simulink model "ssc_auto_ev_20b"  (R2020b)
settings: Solver=VariableStepAuto  StartTime=0.0  StopTime=200  RelTol=1e-3  AbsTol=1e-3
PreLoadFcn:
  | % Simulation parameters
  | dt = 0.01;
  | 
  | % Battery cell parameters
  | ssc_lithium_cell_1RC_ini
  | Nseries = 100;
  | Nparallel = 10;
  | 
  | % Motor parameters
  | max_torque = 220;
  | max_power = 80e3;
  | 
  | % Vehicle parameters
  | vehicle_mass = 4000;
  | wheel_radius = 0.35;
  | area = 5;
  | drag_coefficient = 0.25;
  | air_density = 1.225;
  | gravity = 9.81;
  | rolling_res_ratio = 0.015;
  | 
  | % Differential drive parameters
  | gear_ratio = 12;
  | 
  | % Simplified braking system parameters
  | force_max_pedal = 500;
  | braking_torque_to_pedal_force_ratio = -16;
  | 
  | % Vehicle controller parameters
  | hill_hold_max_speed = 0.5;
  | 
  | % Water properties for cooling circuit
  | load WaterProperties
  | 
  | % Input signals for Signal Editor block
  | load ssc_auto_ev_Inputs
values from neighbouring files (symbols this model uses):
  C1_LUT = [1913.6 4625.7 23306 10736 18036 12251 9022.9 12447 18872 40764 18721 33630 ... (21 elements, 7x3)]    [ssc_auto_ev_param.mat]
  Capacity_LUT = [28.0081 27.625 27.6392]    [ssc_auto_ev_param.mat]
  cell_Cp_heat = 810.5328    [ssc_auto_ev_param.mat]
  cell_mass = 1    [ssc_auto_ev_param.mat]
  Em_LUT = [3.4966 3.5519 3.6183 3.7066 3.9131 4.0748 4.1923 3.5057 3.566 3.6337 3.7127 3.9259 ... (21 elements, 7x3)]    [ssc_auto_ev_param.mat]
  Qe_init = 15.6845    [ssc_auto_ev_param.mat]
  R0_LUT = [0.0117 0.011 0.0114 0.0107 0.0107 0.0113 0.0116 0.0085 0.0085 0.0087 0.0082 0.0083 ... (21 elements, 7x3)]    [ssc_auto_ev_param.mat]
  R1_LUT = [0.0109 0.0069 0.0047 0.0034 0.0033 0.0033 0.0028 0.0029 0.0024 0.0026 0.0016 0.0023 ... (21 elements, 7x3)]    [ssc_auto_ev_param.mat]
  SOC_LUT = [0 0.1 0.25 0.5 0.75 0.9 1]    [ssc_auto_ev_param.mat]
  T_init = 293.15    [ssc_auto_ev_param.mat]
  Temperature_LUT = [278.15 293.15 313.15]    [ssc_auto_ev_param.mat]
undefined symbols (not defined in the file or in its folder): DiscIntNeverNeededParam, K, Lambda, tau, x0
libraries: fl_lib x656, nesl_utility x86, simulink x21, LiBatteryElements_lib x16, SignalEditorBlockLib x4, simulink_extras x4
(part 9 of 13)

== system ssc_auto_ev_20b/Step 3: Ungroup and Redraw/Motor Drive/DC Motor2 ==
  Inertia : fl_lib/Mechanical/Rotational Elements/Inertia  inertia=0.01 kg*m^2  num_ports=foundation.enum.numPorts2.one  w_specify=off  w_priority=High  w=0 rad/s  w_nominal_specify=off  w_nominal_unit=rad/s  w_nominal_value=1  t_specify=off  t_priority=High  t=0 N*m  t_nominal_specify=off  t_nominal_unit=N*m  t_nominal_value=1
      settings: SourceProductBaseCode=PW,SS,VE
  Rotational Electromechanical Converter : fl_lib/Electrical/Electrical Elements/Rotational Electromechanical Converter  K=1 N*m/A  i_specify=off  i_priority=High  i=0 A  i_nominal_specify=off  i_nominal_unit=A  i_nominal_value=1  v_specify=off  v_priority=High  v=0 V  v_nominal_specify=off  v_nominal_unit=V  v_nominal_value=1  t_specify=off  t_priority=High  t=0 N*m  t_nominal_specify=off  t_nominal_unit=N*m  t_nominal_value=1  w_specify=off  w_priority=High  w=0 rad/s  w_nominal_specify=off  w_nominal_unit=rad/s  w_nominal_value=1
      settings: SourceProductBaseCode=PW,SS,VE
  Thermal Resistor : fl_lib/Electrical/Electrical Elements/Thermal Resistor  R0=1 Ohm  T0=298.15 K  alpha=50e-6 1/K  tc=30 s  K_d=100 W/K  T_specify=off  T_priority=High  T=300 K  T_nominal_specify=off  T_nominal_unit=K  T_nominal_value=1
      settings: SourceProductBaseCode=PW,SS,VE  InternalSimscapePortConfiguration="{\"Bottom\":[],\"Left\":[{\"id\":\"H\",\"label\":\"H\",\"type\":\"foundation.thermal.thermal\"},{\"id\":\"p\",\"label\":\"+\",\"type\":\"foundation.electrical.electrical\"}],\"Right\":[{\"id\":\"n\",\"label\":\"-\",\"type\":\"foundation.electrical.electrical\"}],\"Top\":[]}"
  V+ : PMIOPort  Side=Left
  R : PMIOPort  Port=2  Side=Right
  C : PMIOPort  Port=3  Side=Right
  V- : PMIOPort  Port=4  Side=Left
  H : PMIOPort  Port=5  Side=Left
  connections:
  Thermal Resistor/RConn1 -- Rotational Electromechanical Converter/LConn1
  V-/RConn1 -- Rotational Electromechanical Converter/RConn1
  Thermal Resistor/LConn2 -- V+/RConn1
  Rotational Electromechanical Converter/LConn2 -- Inertia/LConn1 -- R/RConn1
  Rotational Electromechanical Converter/RConn2 -- C/RConn1
  H/RConn1 -- Thermal Resistor/LConn1

== system ssc_auto_ev_20b/Step 3: Ungroup and Redraw/Motor Drive/Motor Torque Controller 1 (System-Level Representation) ==
  Controlled Current Source : fl_lib/Electrical/Electrical Sources/Controlled Current Source
      settings: SourceProductBaseCode=PW,SS,VE
  +1 : PMIOPort  Side=Right
  +2 : PMIOPort  Port=2  Side=Left
  -1 : PMIOPort  Port=3  Side=Right
  -2 : PMIOPort  Port=4  Side=Left
  iRef : PMIOPort  Port=5  Side=Left
  connections:
  iRef/RConn1 -- Controlled Current Source/RConn1
  -2/RConn1 -- -1/RConn1
  Controlled Current Source/LConn1 -- +2/RConn1
  Controlled Current Source/RConn2 -- +1/RConn1

== system ssc_auto_ev_20b/Step 3: Ungroup and Redraw/Motor Drive/Motor Torque Controller 1 (System-Level Representation)1 ==
  Controlled Current Source : fl_lib/Electrical/Electrical Sources/Controlled Current Source
      settings: SourceProductBaseCode=PW,SS,VE
  +1 : PMIOPort  Side=Right
  +2 : PMIOPort  Port=2  Side=Left
  -1 : PMIOPort  Port=3  Side=Right
  -2 : PMIOPort  Port=4  Side=Left
  iRef : PMIOPort  Port=5  Side=Left
  connections:
  Controlled Current Source/RConn2 -- +1/RConn1
  Controlled Current Source/LConn1 -- +2/RConn1
  -2/RConn1 -- -1/RConn1
  iRef/RConn1 -- Controlled Current Source/RConn1

== system ssc_auto_ev_20b/Step 3: Ungroup and Redraw/Motor Drive/Sensing wMotor ==
  PS-Simulink Converter : nesl_utility/PS-Simulink Converter  PhysicalDomain=network_engine_domain  SubClassName=ps_output  LeftPortType=input  RightPortType=output  PseudoPeriodic=off  Frequencies=[]  Unit=rad/s  AffineConversion=off
      settings: SourceProductBaseCode=SS,PW,VE
  PS : PMIOPort  Side=Left
  SL : Outport  VectorParamsAs1DForOutWhenUnconnected=off
  wires:
  PS-Simulink Converter/1 -> SL/1
  connections:
  PS/RConn1 -- PS-Simulink Converter/LConn1

== system ssc_auto_ev_20b/Step 3: Ungroup and Redraw/Port 1 Interface/Interface ==
  through1 : Inport
  through2 : Inport  Port=2
  Continuous : Subsystem  VariantControl=Continuous
  Discrete : Subsystem  VariantControl=Discrete
  across2 : Outport
  across1 : Outport  Port=2

== system ssc_auto_ev_20b/Step 3: Ungroup and Redraw/Port 1 Interface1/Interface ==
  through1 : Inport
  through2 : Inport  Port=2
  Continuous : Subsystem  VariantControl=Continuous
  Discrete : Subsystem  VariantControl=Discrete
  across2 : Outport
  across1 : Outport  Port=2

== system ssc_auto_ev_20b/Step 3: Ungroup and Redraw/Port 1 Interface2/Interface ==
  through1 : Inport
  through2 : Inport  Port=2
  Continuous : Subsystem  VariantControl=Continuous
  Discrete : Subsystem  VariantControl=Discrete
  across2 : Outport
  across1 : Outport  Port=2

== system ssc_auto_ev_20b/Step 3: Ungroup and Redraw/Port 1 Interface3/Interface ==
  through1 : Inport
  across2 : Inport  Port=2
  Continuous : Subsystem  VariantControl=Continuous
  Discrete : Subsystem  VariantControl=Discrete
  through2 : Outport
  across1 : Outport  Port=2

== system ssc_auto_ev_20b/Step 3: Ungroup and Redraw/Vehicle Dynamics/Brake Torque ==
  Pedal : Inport
  Force for max pedal deflection : Gain  Gain=force_max_pedal
  Ideal Torque Source : fl_lib/Mechanical/Mechanical Sources/Ideal Torque Source
      settings: SourceProductBaseCode=PW,SS,VE
  MRRef : fl_lib/Mechanical/Rotational Elements/Mechanical Rotational Reference
      settings: SourceProductBaseCode=PW,SS,VE
  Motion Sensor : fl_lib/Mechanical/Mechanical Sensors/Ideal Rotational Motion Sensor  wrap_angle=simscape.enum.onoff.off  offset=0 rad
      settings: SourceProductBaseCode=PW,SS,VE
  PS Product : fl_lib/Physical Signals/Functions/PS Product
      settings: SourceProductBaseCode=PW,SS,VE
  Simulink-PS Converter1 : nesl_utility/Simulink-PS Converter  PhysicalDomain=network_engine_domain  SubClassName=ps_input  LeftPortType=input  RightPortType=output  PseudoPeriodic=off  Frequencies=[]  NoiseDistribution=none  NoiseParameters=[]  Unit=N*m  AffineConversion=off  FilteringAndDerivatives=zero  SimscapeFilterOrder=1  InputFilterTimeConstant=0.001  UdotUserProvided=1
      settings: SourceProductBaseCode=SS,PW,VE
  Smooth Sign : Subsystem
  Torque per unit brake pedal force : Gain  Gain=braking_torque_to_pedal_force_ratio
  R : PMIOPort  Side=Right
  wires:
  Torque per unit brake pedal force/1 -> Simulink-PS Converter1/1
  Pedal/1 -> Force for max pedal deflection/1
  Force for max pedal deflection/1 -> Torque per unit brake pedal force/1
  connections:
  Smooth Sign/RConn1 -- PS Product/LConn1
  Motion Sensor/RConn1 -- MRRef/LConn1 -- Ideal Torque Source/RConn2
  Ideal Torque Source/LConn1 -- Motion Sensor/LConn1 -- R/RConn1
  PS Product/RConn1 -- Ideal Torque Source/RConn1
  PS Product/LConn2 -- Simulink-PS Converter1/RConn1
  Smooth Sign/LConn1 -- Motion Sensor/RConn2

== system ssc_auto_ev_20b/Step 3: Ungroup and Redraw/Vehicle Dynamics/Drag and Gravity ==
  beta : Inport
  vW : Inport  Port=2
  " M*g " : fl_lib/Physical Signals/Functions/PS Gain  gain=vehicle_mass*gravity kg*m/s^2
      settings: SourceProductBaseCode=PW,SS,VE
  " tanh(u) " : fl_lib/Physical Signals/Functions/PS Math Function  fcn_choice=foundation.enum.math_function.tanh
      settings: SourceProductBaseCode=PW,SS,VE
  -1 : fl_lib/Physical Signals/Functions/PS Gain  gain=-1
      settings: SourceProductBaseCode=PW,SS,VE
  0.5*Cd*density*area : fl_lib/Physical Signals/Functions/PS Gain  gain=0.5*drag_coefficient*air_density*area kg/m^3*m^2
      settings: SourceProductBaseCode=PW,SS,VE
  1s/m : fl_lib/Physical Signals/Functions/PS Gain  gain=1 1/(m/s)
      settings: SourceProductBaseCode=PW,SS,VE
  M*g : fl_lib/Physical Signals/Functions/PS Gain  gain=vehicle_mass*gravity kg*m/s^2
      settings: SourceProductBaseCode=PW,SS,VE
  PS Add : fl_lib/Physical Signals/Functions/PS Add
      settings: SourceProductBaseCode=PW,SS,VE
  PS Gain : fl_lib/Physical Signals/Functions/PS Gain  gain=1 1/(m/s)
      settings: SourceProductBaseCode=PW,SS,VE
  PS Product : fl_lib/Physical Signals/Functions/PS Product
      settings: SourceProductBaseCode=PW,SS,VE
  PS Product2 : fl_lib/Physical Signals/Functions/PS Product
      settings: SourceProductBaseCode=PW,SS,VE
  PS Subtract : fl_lib/Physical Signals/Functions/PS Subtract
      settings: SourceProductBaseCode=PW,SS,VE
  Rolling resistance (fraction of normal force) : fl_lib/Physical Signals/Functions/PS Gain  gain=rolling_res_ratio
      settings: SourceProductBaseCode=PW,SS,VE
  Simulink-PS Converter2 : nesl_utility/Simulink-PS Converter  PhysicalDomain=network_engine_domain  SubClassName=ps_input  LeftPortType=input  RightPortType=output  PseudoPeriodic=off  Frequencies=[]  NoiseDistribution=none  NoiseParameters=[]  Unit=m/s  AffineConversion=off  FilteringAndDerivatives=zero  SimscapeFilterOrder=1  InputFilterTimeConstant=0.001  UdotUserProvided=1
      settings: SourceProductBaseCode=SS,PW,VE
  Simulink-PS Converter3 : nesl_utility/Simulink-PS Converter  PhysicalDomain=network_engine_domain  SubClassName=ps_input  LeftPortType=input  RightPortType=output  PseudoPeriodic=off  Frequencies=[]  NoiseDistribution=none  NoiseParameters=[]  Unit=deg  AffineConversion=off  FilteringAndDerivatives=zero  SimscapeFilterOrder=1  InputFilterTimeConstant=0.001  UdotUserProvided=1
      settings: SourceProductBaseCode=SS,PW,VE
  cos(u) : fl_lib/Physical Signals/Functions/PS Math Function  fcn_choice=foundation.enum.math_function.cos
      settings: SourceProductBaseCode=PW,SS,VE
  sin(u) : fl_lib/Physical Signals/Functions/PS Math Function  fcn_choice=foundation.enum.math_function.sin
      settings: SourceProductBaseCode=PW,SS,VE
  tanh(u) : fl_lib/Physical Signals/Functions/PS Math Function  fcn_choice=foundation.enum.math_function.tanh
      settings: SourceProductBaseCode=PW,SS,VE
  u^2 : fl_lib/Physical Signals/Functions/PS Math Function  fcn_choice=foundation.enum.math_function.square
      settings: SourceProductBaseCode=PW,SS,VE
  vV : PMIOPort  Side=Left
  F : PMIOPort  Port=2  Side=Left
  F2 : PMIOPort  Port=3  Side=Left
  wires:
  beta/1 -> Simulink-PS Converter3/1
  vW/1 -> Simulink-PS Converter2/1
  connections:
  " M*g "/LConn1 -- cos(u)/RConn1
  M*g/LConn1 -- sin(u)/RConn1
  Rolling resistance (fraction of normal force)/LConn1 -- " M*g "/RConn1
  M*g/RConn1 -- PS Add/LConn1
  sin(u)/LConn1 -- Simulink-PS Converter3/RConn1 -- cos(u)/LConn1
  PS Product2/LConn2 -- 0.5*Cd*density*area/RConn1
  " tanh(u) "/LConn1 -- PS Gain/RConn1
  0.5*Cd*density*area/LConn1 -- u^2/RConn1
  " tanh(u) "/RConn1 -- PS Product2/LConn1
  u^2/LConn1 -- PS Subtract/RConn1 -- PS Gain/LConn1
  tanh(u)/LConn1 -- 1s/m/RConn1
  PS Product/LConn1 -- tanh(u)/RConn1
  -1/RConn1 -- F2/RConn1
  PS Add/RConn1 -- -1/LConn1
  PS Product/RConn1 -- PS Add/LConn2
  PS Product/LConn2 -- Rolling resistance (fraction of normal force)/RConn1
  PS Product2/RConn1 -- F/RConn1
  Simulink-PS Converter2/RConn1 -- PS Subtract/LConn2
  PS Subtract/LConn1 -- 1s/m/LConn1 -- vV/RConn1

== system ssc_auto_ev_20b/Step 3: Ungroup and Redraw/Vehicle Dynamics/Sensing Speed ==
  MTRef : fl_lib/Mechanical/Translational Elements/Mechanical Translational Reference
      settings: SourceProductBaseCode=PW,SS,VE
  Motion Sensor : fl_lib/Mechanical/Mechanical Sensors/Ideal Translational Motion Sensor  offset=0 m
      settings: SourceProductBaseCode=PW,SS,VE
  R : PMIOPort  Side=Left
  w : PMIOPort  Port=2  Side=Right
  connections:
  R/RConn1 -- Motion Sensor/LConn1
  MTRef/LConn1 -- Motion Sensor/RConn1
  Motion Sensor/RConn2 -- w/RConn1

== system ssc_auto_ev_20b/Step 3: Ungroup and Redraw/Vehicle Control/Cruise Control ==
  Enable : Inport
  Disable : Inport  Port=2
  wMeas : Inport  Port=3
  Brake sw : Inport  Port=4
  Capture speed : Subsystem  TreatAsAtomicUnit=on
  Data Type Conversion1 : DataTypeConversion  OutDataTypeStr=boolean
  J-K Flip-Flop : simulink_extras/Flip Flops/J-K Flip-Flop  initial_condition=0
  Logical Operator : Logic  Operator=OR  AllPortsSameDT=off  OutDataTypeStr=boolean
  Pulse Generator : DiscretePulseGenerator  Period=10  PulseWidth=5  SampleTime=0.01
  Speed Controller : Subsystem  mask(P+I motor speed controller){Kp=100, Ki=100, trqMax=max_torque, ts=dt}
      mask prompts: Kp "Proportional gain (Nm/(rad/s))"; Ki "Integral gain (Nm/rad)"; trqMax "Maximum torque demand"; ts "Sample time"
      mask help: Inputs wRef and wMeas are the demanded rotor speed and measured rotor speed in rad/s. The controller output is a torque demand in Nm.
  Terminator : Terminator
  trqRef : Outport  VectorParamsAs1DForOutWhenUnconnected=off
  Enabled : Outport  Port=2  VectorParamsAs1DForOutWhenUnconnected=off
  wires:
  Enable/1 -> Data Type Conversion1/1
  Pulse Generator/1 -> J-K Flip-Flop/2
  Disable/1 -> Logical Operator/1
  Speed Controller/1(trqRef) -> trqRef/1
  Brake sw/1 -> Logical Operator/2
  wMeas/1 -> Capture speed/1(In1), Speed Controller/2(wMeas)
  Logical Operator/1 -> J-K Flip-Flop/3
  J-K Flip-Flop/1 -> Enabled/1, Capture speed/Trigger
  Data Type Conversion1/1 -> J-K Flip-Flop/1
  J-K Flip-Flop/2 -> Terminator/1
  Capture speed/1(Out1) -> Speed Controller/1(wRef)

== system ssc_auto_ev_20b/Step 3: Ungroup and Redraw/Vehicle Control/Feedforward term for regenerative braking on downhill ==
  Inclin. : Inport
  " M " : Gain  Gain=vehicle_mass
  1/ratio : Gain  Gain=1/gear_ratio
  Two motors : Gain  Gain=0.5
  Wheel radius : Gain  Gain=wheel_radius
  "[-inf,0]" : Saturate  UpperLimit=0  LowerLimit=-inf
  Feedfwd trq : Outport  VectorParamsAs1DForOutWhenUnconnected=off
  wires:
  Two motors/1 -> Feedfwd trq/1
  1/ratio/1 -> Two motors/1  "Motor torque"
  "[-inf,0]"/1 -> " M "/1
  Inclin./1 -> "[-inf,0]"/1
  " M "/1 -> Wheel radius/1
  Wheel radius/1 -> 1/ratio/1  "Wheel torque"

== system ssc_auto_ev_20b/Step 3: Ungroup and Redraw/Vehicle Control/Max Power ==
  Vspd : Inport
  Abs : Abs
  Constant : Constant
  Math Function : Math  Operator=reciprocal  SignedPower=on  SaturateOnIntegerOverflow=on
  Prevent divide by zero : Switch  Criteria=u2 > Threshold  Threshold=1
  max_power : Gain  Gain=max_power
  Max Power : Outport  VectorParamsAs1DForOutWhenUnconnected=off
  wires:
  Prevent divide by zero/1 -> Math Function/1
  Constant/1 -> Prevent divide by zero/3
  Abs/1 -> Prevent divide by zero/2, Prevent divide by zero/1
  Math Function/1 -> max_power/1
  max_power/1 -> Max Power/1
  Vspd/1 -> Abs/1

== system ssc_auto_ev_20b/Step 3: Ungroup and Redraw/Vehicle Control/Torque Demand Management ==
  Brake : Inport
  Throttle : Inport  Port=2
  wMeas : Inport  Port=3
  FFbrake : Inport  Port=4
  1/ratio : Gain  Gain=1/gear_ratio
  Disable braking at low and negative speeds : Lookup_n-D  NumberOfTableDimensions=1  BreakpointsForDimension1=[-100 -1 0 5 10 100]  Table=[0 0 0 0 1 1]  InternalRulePriority=Speed  RndMeth=Simplest  InputSameDT=on
  Disable braking at low and negative speeds1 : Lookup_n-D  NumberOfTableDimensions=1  BreakpointsForDimension1=[-100 -1 0 5 10 100]  Table=[0 0 0 0 1 1]  InternalRulePriority=Speed  RndMeth=Simplest  InputSameDT=on
  Force for max pedal deflection : Gain  Gain=force_max_pedal
  Max torque demand : Gain  Gain=max_torque
  Motor torque limits2 : Saturate  UpperLimit=max_torque  LowerLimit=-max_torque
  Product : Product
  Product1 : Product
  Sum : Sum  Inputs=|++
  Sum1 : Sum  Inputs=|++
  Torque per unit brake pedal force : Gain  Gain=braking_torque_to_pedal_force_ratio
  Two motors : Gain  Gain=1/2
  wMeas1 : InportShadow  Port=3
  Dem trq : Outport  VectorParamsAs1DForOutWhenUnconnected=off
  wires:
  Motor torque limits2/1 -> Dem trq/1
  Sum1/1 -> Motor torque limits2/1
  Product1/1 -> Sum1/2
  wMeas1/1 -> Disable braking at low and negative speeds1/1
  Disable braking at low and negative speeds1/1 -> Product1/2
  FFbrake/1 -> Product1/1
  Disable braking at low and negative speeds/1 -> Product/2
  Sum/1 -> Sum1/1
  Max torque demand/1 -> Sum/1
  Brake/1 -> Force for max pedal deflection/1
  Throttle/1 -> Max torque demand/1
  Torque per unit brake pedal force/1 -> 1/ratio/1
  1/ratio/1 -> Two motors/1
  Force for max pedal deflection/1 -> Torque per unit brake pedal force/1
  wMeas/1 -> Disable braking at low and negative speeds/1
  Product/1 -> Sum/2
  Two motors/1 -> Product/1

== system ssc_auto_ev_20b/Step 4: Deployment Model/Battery @50Hz/Battery ==
  note: Scale up voltage drop to total
      | of Ns series-connected cells
  Controlled Voltage Source : fl_lib/Electrical/Electrical Sources/Controlled Voltage Source
      settings: SourceProductBaseCode=PW,SS,VE
  Electric and Thermal Model : Subsystem  Tag=PublishSubsystem
  Nseries-1 : fl_lib/Physical Signals/Functions/PS Gain  gain=Nseries-1
      settings: SourceProductBaseCode=PW,SS,VE
  PS Terminator : fl_lib/Physical Signals/Sinks/PS Terminator
      settings: SourceProductBaseCode=PW,SS,VE
  Temperature Sensor : fl_lib/Thermal/Thermal Sensors/Temperature Sensor
      settings: SourceProductBaseCode=PW,SS,VE
  Thermal Reference : fl_lib/Thermal/Thermal Elements/Thermal Reference
      settings: SourceProductBaseCode=PW,SS,VE
  Voltage Sensor : fl_lib/Electrical/Electrical Sensors/Voltage Sensor
      settings: SourceProductBaseCode=PW,SS,VE
  + : PMIOPort  Tag=PMCPort  Side=Right
  H : PMIOPort  Tag=PMCPort  Port=2  Side=Left
  - : PMIOPort  Tag=PMCPort  Port=3  Side=Left
  connections:
  PS Terminator/LConn1 -- Temperature Sensor/RConn2
  Temperature Sensor/RConn1 -- Thermal Reference/LConn1
  Controlled Voltage Source/RConn2 -- -/RConn1
  Nseries-1/RConn1 -- Controlled Voltage Source/RConn1
  +/RConn1 -- Electric and Thermal Model/RConn1 -- Voltage Sensor/LConn1
  Nseries-1/LConn1 -- Voltage Sensor/RConn1
  Electric and Thermal Model/RConn2 -- Voltage Sensor/RConn2 -- Controlled Voltage Source/LConn1
  Electric and Thermal Model/LConn1 -- Temperature Sensor/LConn1 -- H/RConn1

== system ssc_auto_ev_20b/Step 4: Deployment Model/Battery @50Hz/Port 1 Interface ==
  heat flow : Inport
  Controlled Temperature Source : fl_lib/Thermal/Thermal Sources/Controlled Temperature Source
      settings: SourceProductBaseCode=PW,SS,VE
  Heat Flow Rate Sensor : fl_lib/Thermal/Thermal Sensors/Heat Flow Rate Sensor
      settings: SourceProductBaseCode=PW,SS,VE
  Interface : Subsystem  Variant=on  VariantControlMode=label  VariantControl=Variant1  LabelModeActiveChoice=Discrete
      settings: PortSchema="{\"entries\":[{\"content\":{\"sides\":[{\"content\":{\"connectorIds\":[\"In1\",\"Out2\"]},\"type\":\"ConnectorPlacement.EquallySpacedRectSide\",\"uuid\":\"aa56821c-7799-44e3-b228-553c5b43a68d\"},{\"content\":{\"connectorIds\":[\"In2\",\"Out1\"],\"side\":\"RIGHT\"},\"type\":\"ConnectorPlacement.EquallySpacedRectSide\",\"uuid\":\"8658dee5-55e2-4f33-bdec-e6600ce27fc1\"},{\"content\":{\"connectorIds\":[],\"side\":\"TOP\"},\"type\":\"ConnectorPlacement.EquallySpacedRectSide\",\"uuid\":\"2effe9c6-8e61-4f0c-a39b-329d9ffc707d\"}]},\"type\":\"ConnectorPlacement.EquallySpacedConnector\",\"uuid\":\"c8fc8444-dfc7-49a5-9550-b957635f7d8f\"}],\"packageUris\":[\"http://schema.mathworks.com/mf0/Connector/R2020b\"],\"version\":\"1.0\"}"
  T1 : nesl_utility/Simulink-PS Converter  PhysicalDomain=network_engine_domain  SubClassName=ps_input  LeftPortType=input  RightPortType=output  PseudoPeriodic=off  Frequencies=[]  NoiseDistribution=none  NoiseParameters=[]  Unit=K  AffineConversion=off  FilteringAndDerivatives=provide  SimscapeFilterOrder=1  InputFilterTimeConstant=0.001  UdotUserProvided=0
      settings: SourceProductBaseCode=SS,PW,VE
  Thermal Reference : fl_lib/Thermal/Thermal Elements/Thermal Reference
      settings: SourceProductBaseCode=PW,SS,VE
  q1 : nesl_utility/PS-Simulink Converter  PhysicalDomain=network_engine_domain  SubClassName=ps_output  LeftPortType=input  RightPortType=output  PseudoPeriodic=off  Frequencies=[]  Unit=W  AffineConversion=off
      settings: SourceProductBaseCode=SS,PW,VE
  1 : PMIOPort  Side=Left
  temperature : Outport
  wires:
  Interface/1(across2) -> temperature/1
  q1/1 -> Interface/1(through1)
  heat flow/1 -> Interface/2(through2)
  Interface/2(across1) -> T1/1
  connections:
  Heat Flow Rate Sensor/RConn2 -- Controlled Temperature Source/LConn1
  Heat Flow Rate Sensor/LConn1 -- 1/RConn1
  q1/LConn1 -- Heat Flow Rate Sensor/RConn1
  Thermal Reference/LConn1 -- Controlled Temperature Source/RConn2
  Controlled Temperature Source/RConn1 -- T1/RConn1

== system ssc_auto_ev_20b/Step 4: Deployment Model/Battery @50Hz/Port 2 Interface3 ==
  current : Inport
  Controlled Current Source : fl_lib/Electrical/Electrical Sources/Controlled Current Source
      settings: SourceProductBaseCode=PW,SS,VE
  Electrical Reference : fl_lib/Electrical/Electrical Elements/Electrical Reference
      settings: SourceProductBaseCode=PW,SS,VE
  Electrical Reference1 : fl_lib/Electrical/Electrical Elements/Electrical Reference
      settings: SourceProductBaseCode=PW,SS,VE
  In : nesl_utility/Simulink-PS Converter  PhysicalDomain=network_engine_domain  SubClassName=ps_input  LeftPortType=input  RightPortType=output  PseudoPeriodic=off  Frequencies=[]  NoiseDistribution=none  NoiseParameters=[]  Unit=A  AffineConversion=off  FilteringAndDerivatives=zero  SimscapeFilterOrder=1  InputFilterTimeConstant=0.001  UdotUserProvided=1
      settings: SourceProductBaseCode=SS,PW,VE
  Vn : nesl_utility/PS-Simulink Converter  PhysicalDomain=network_engine_domain  SubClassName=ps_output  LeftPortType=input  RightPortType=output  PseudoPeriodic=off  Frequencies=[]  Unit=V  AffineConversion=off
      settings: SourceProductBaseCode=SS,PW,VE
  Voltage Sensor : fl_lib/Electrical/Electrical Sensors/Voltage Sensor
      settings: SourceProductBaseCode=PW,SS,VE
  2 : PMIOPort  Side=Right
  voltage : Outport
  wires:
  current/1 -> In/1
  Vn/1 -> voltage/1
  connections:
  In/RConn1 -- Controlled Current Source/RConn1
  Controlled Current Source/LConn1 -- Electrical Reference/LConn1
  Voltage Sensor/RConn1 -- Vn/LConn1
  2/RConn1 -- Controlled Current Source/RConn2 -- Voltage Sensor/LConn1
  Electrical Reference1/LConn1 -- Voltage Sensor/RConn2

== system ssc_auto_ev_20b/Step 4: Deployment Model/Control @100Hz/Driver and Environment ==
  Bus : Subsystem
  Bus Creator : BusCreator  Inputs=5
  Inclinometer : Subsystem
  Inputs : SignalEditorBlockLib/Signal Editor  FileName=ssc_auto_ev_Inputs.mat  ActiveScenario=Test_1  ActiveSignal=Env (deg C)  IsBus=off  OutputBusObjectStr=Bus: BusObject  SampleTime=0.01  OutputAfterFinalValue=Extrapolation  Unit=inherit  PreserveSignalName=on
  ZOH/{2..3,5..7} (5 alike) : ZeroOrderHold  SampleTime=dt
  Veh : Outport
  ECU : Outport  Port=2
  Env : Outport  Port=3
  wires:
  ? -> Bus/3(Br), ZOH/5/1
  ZOH/6/1 -> Bus Creator/1  "Incline"
  ZOH/7/1 -> Bus Creator/5  "Cruise disable"
  ZOH/3/1 -> Bus Creator/4  "Cruise enable"
  ZOH/2/1 -> Bus Creator/3  "Throttle"
  ZOH/5/1 -> Bus Creator/2  "Brake pedal"
  Bus Creator/1 -> ECU/1
  Bus/1(b) -> Veh/1
  ? -> Env/1
  ? -> ZOH/7/1
  Inputs/1 -> Inclinometer/1(a), Bus/1(In)
  ? -> ZOH/3/1
  ? -> ZOH/2/1
  Inclinometer/1(y) -> ZOH/6/1
  ? -> Bus/2(Wi)

== system ssc_auto_ev_20b/Step 4: Deployment Model/Control @100Hz/Vehicle Control ==
  ECU : Inport
  wMeas : Inport  Port=2
  -1 : Gain  Gain=-1
  1/Kt : Gain  Gain=1/1
  Bus Selector : BusSelector  OutputSignals=Cruise enable,Cruise disable,Brake pedal,Throttle,Incline
  Compare To Constant : simulink/Logic and Bit Operations/Compare To Constant  relop=>  const=0  OutDataTypeStr=boolean
  Cruise Control : Subsystem
  Feedforward term for regenerative braking on downhill : Subsystem
  Max Power : Subsystem
  Power limits : simulink/Discontinuities/Saturation Dynamic  OutMin=[]  OutMax=[]  OutDataTypeStr=Inherit: Same as second input  OutDataType=fixdt(1, 16)  OutScaling=2^-10  DoSatur=off
  Switch between torque control and speed control : Switch  Criteria=u2 > Threshold
  Torque limits : Saturate  UpperLimit=max_torque  LowerLimit=-max_torque
  Torque Demand Management : Subsystem
  iRef : Outport  VectorParamsAs1DForOutWhenUnconnected=off
  wires:
  Feedforward term for regenerative braking on downhill/1(Feedfwd trq) -> Torque Demand Management/4(FFbrake)
  1/Kt/1 -> iRef/1
  ECU/1 -> Bus Selector/1
  Cruise Control/2(Enabled) -> Switch between torque control and speed control/2
  Torque Demand Management/1(Dem trq) -> Switch between torque control and speed control/3
  Switch between torque control and speed control/1 -> Torque limits/1
  Bus Selector/1 -> Cruise Control/1(Enable)  "<Cruise enable>"
  wMeas/1 -> Max Power/1(Vspd), Cruise Control/3(wMeas), Torque Demand Management/3(wMeas)
  Cruise Control/1(trqRef) -> Switch between torque control and speed control/1
  Bus Selector/2 -> Cruise Control/2(Disable)  "<Cruise disable>"
  Compare To Constant/1 -> Cruise Control/4(Brake sw)
  Bus Selector/4 -> Torque Demand Management/2(Throttle)  "<Throttle>"
  Bus Selector/3 -> Torque Demand Management/1(Brake), Compare To Constant/1  "<Brake pedal>"
  Bus Selector/5 -> Feedforward term for regenerative braking on downhill/1(Inclin.)  "<Incline>"
  Torque limits/1 -> Power limits/2
  Power limits/1 -> 1/Kt/1
  -1/1 -> Power limits/3
  Max Power/1(Max Power) -> -1/1, Power limits/1

== system ssc_auto_ev_20b/Step 4: Deployment Model/Thermal @20Hz/Cooling System ==
  note: Battery Heat Exchanger
  note: Radiator
  " Heat Exchanger Characteristic" : Subsystem
  Convection Battery-Env : fl_lib/Thermal/Thermal Elements/Convective Heat Transfer  area=cell_area m^2  heat_tr_coeff=h_conv W/(m^2 * K)  T_specify=off  T_priority=High  T=0 K  T_nominal_specify=off  T_nominal_unit=K  T_nominal_value=1  Q_specify=off  Q_priority=High  Q=0 J/s  Q_nominal_specify=off  Q_nominal_unit=J/s  Q_nominal_value=1
      settings: SourceProductBaseCode=PW,SS,VE
  Expansion Tank : Subsystem
  Heat Exchanger Characteristic : Subsystem
  Hose Radiator : fl_lib/Thermal Liquid/Elements/Pipe (TL)  length=2000 mm  area=pi*25^2 mm^2  Dh=50 mm  length_add=500 mm  roughness=1.5e-5 m  Re_lam=2e+3  Re_tur=4e+3  shape_factor=64  Nu_lam=3.66  dynamic_compressibility=1  inertia=0  p0=1 atm  T0=20 degC  mdot0=0.1 kg/s
      settings: SourceProductBaseCode=PW,SS,VE
  Hose Inlet : fl_lib/Thermal Liquid/Elements/Pipe (TL)  length=500 mm  area=pi*25^2 mm^2  Dh=50 mm  length_add=500 mm  roughness=1.5e-5 m  Re_lam=2e+3  Re_tur=4e+3  shape_factor=64  Nu_lam=3.66  dynamic_compressibility=1  inertia=0  p0=1 atm  T0=20 degC  mdot0=0.1 kg/s
      settings: SourceProductBaseCode=PW,SS,VE
  Hose Outlet : fl_lib/Thermal Liquid/Elements/Pipe (TL)  length=500 mm  area=pi*25^2 mm^2  Dh=50 mm  length_add=500 mm  roughness=1.5e-5 m  Re_lam=2e+3  Re_tur=4e+3  shape_factor=64  Nu_lam=3.66  dynamic_compressibility=1  inertia=0  p0=1 atm  T0=20 degC  mdot0=0.1 kg/s
      settings: SourceProductBaseCode=PW,SS,VE
  Insulator Inlet Hose : fl_lib/Thermal/Thermal Elements/Perfect Insulator  T_specify=off  T_priority=High  T=0 K  T_nominal_specify=off  T_nominal_unit=K  T_nominal_value=1
      settings: SourceProductBaseCode=PW,SS,VE
  Insulator Outlet Hose : fl_lib/Thermal/Thermal Elements/Perfect Insulator  T_specify=off  T_priority=High  T=0 K  T_nominal_specify=off  T_nominal_unit=K  T_nominal_value=1
      settings: SourceProductBaseCode=PW,SS,VE
  PS Terminator : fl_lib/Physical Signals/Sinks/PS Terminator
      settings: SourceProductBaseCode=PW,SS,VE
  Pipe : fl_lib/Thermal Liquid/Elements/Pipe (TL)  length=400 mm  area=pi*25^2 mm^2  Dh=50 mm  length_add=500 mm  roughness=1.5e-5 m  Re_lam=2e+3  Re_tur=4e+3  shape_factor=64  Nu_lam=3.66  dynamic_compressibility=1  inertia=0  p0=1 atm  T0=20 degC  mdot0=0.1 kg/s
      settings: SourceProductBaseCode=PW,SS,VE
  Pump : fl_lib/Thermal Liquid/Sources/Mass Flow Rate Source (TL)  commanded_mass_flow=0.2 kg/s  area=pi*25^2 mm^2
      settings: SourceProductBaseCode=PW,SS,VE  InternalSimscapePortConfiguration="{\"Bottom\":[],\"Left\":[{\"id\":\"A\",\"label\":\"A\",\"type\":\"foundation.thermal_liquid.thermal_liquid\"}],\"Right\":[{\"id\":\"B\",\"label\":\"B\",\"type\":\"foundation.thermal_liquid.thermal_liquid\"}],\"Top\":[]}"
  Sensing Inlet Temperature : Subsystem
      mask Display: disp('T');
  Sensing Temperature : Subsystem
      mask Display: disp('T')
  Thermal Liquid Settings (TL) : fl_lib/Thermal Liquid/Utilities/Thermal Liquid Settings (TL)  table_dimensions=0  T_TLU=T K  p_TLU=p Pa  p_atm=1 atm  pT_region_flag=0  T_min=273.16 K  T_max=373.16 K  p_min=0.1 bar  p_max=500 bar  T_min_1D=273.16 K  T_max_1D=373.16 K  p_min_1D=0.01 MPa  p_max_1D=50 MPa  pT_validity_TLU=ones(11, 12)  rho_parameterization_2D=1  rho_parameterization_1D=1  rho_TLU=rho kg/m^3  beta_TLU=beta Pa  alpha_TLU=alpha 1/K  rho_TLU_2=[999.7973, 999.8431, 1002.3216, 1004.8218, 1007.293, 1009.7358, 1012.1506, 1014.5379, 1016.8979, 1019.2311, 1021.538, 1023.8188; 999.6579, 999.7009, 1002.0303, 1004.382, 1006.7084, 1009.0101, 1011.2874, 1013.5407, 1015.7703, 1017.9766, 1020.1599, 1022.3206; 998.1632, 998.2045, 1000.4375, 1002.6924, 1004.9239, 1007.1324, 1009.3183, 1011.4819, 1013.6236, 1015.7438, 1017.8428, 1019.921; 995.6057, 995.6458, 997.81864, 1000.0128, 1002.1841, 1004.3332, 1006.4603, 1008.566, 1010.6505, 1012.7144, 1014.758, 1016.7815; 992.1724, 992.2119, 994.35133, 996.5113, 998.6484, 1000.7633, 1002.8563, 1004.928, 1006.9788, 1009.009, 1011.0192, 1013.0097; 988.02, 988.0299, 990.15684, 992.3035, 994.4268, 996.5273, 998.6056, 1000.6622, 1002.6976, 1004.7123, 1006.7067, 1008.6813; 983.18, 983.1901, 985.3217, 987.4721, 989.5983, 991.7008, 993.7803, 995.8374, 997.8726, 999.8864, 1001.8795, 1003.8522; 977.75, 977.7583, 979.9094, 982.0783, 984.2216, 986.34, 988.4343, 990.505, 992.5529, 994.5786, 996.5825, 998.5654; 971.77, 971.7836, 973.96734, 976.1678, 978.3409, 980.4876, 982.6087, 984.7049, 986.7768, 988.8254, 990.8511, 992.8545; 965.26, 965.3023, 967.53107, 969.7753, 971.9901, 974.1764, 976.3354, 978.4676, 980.5741, 982.6556, 984.7129, 986.7465; 958.62, 958.6315, 960.627, 962.9267, 965.1944, 967.4314, 969.6387, 971.8173, 973.9681, 976.0921, 978.19, 980.2628] kg/m^3  rho_ref_3=998.21 kg/m^3  T_ref_3=293.16 K  p_ref_3=0.101325 MPa  beta_const_3=2.1791 GPa  alpha_const_3=2.0691e-4 1/K  rho_TLU_4=[999.84; 999.7; 998.2; 995.65; 992.21; 988.03; 983.19; 977.76; 971.78; 965.3; 958.8] kg/m^3  beta_const_4=2.1791 GPa  p_ref_4=0.101325 MPa  rho_ref_5=998.21 kg/m^3  T_ref_5=293.16 K  p_ref_5=0.101325 MPa  beta_const_5=2.1791 GPa  alpha_const_5=2.0691e-4 1/K  u_parameterization_2D=1  u_parameterization_1D=1  u_TLU=u J/g  cp_TLU=Cp J/K/g  u_TLU_2=[.0002, .0018, .086, .1588, .219, .267, .3034, .3288, .3436, .3483, .3435, .3294; 42.062, 42.06, 41.935, 41.804, 41.668, 41.527, 41.382, 41.233, 41.081, 40.924, 40.763, 40.599; 83.953, 83.948, 83.651, 83.349, 83.049, 82.749, 82.451, 82.153, 81.856, 81.56, 81.265, 80.971; 125.77, 125.76, 125.31, 124.86, 124.41, 123.97, 123.53, 123.1, 122.68, 122.25, 121.84, 121.42; 167.57, 167.56, 166.96, 166.37, 165.79, 165.21, 164.65, 164.09, 163.54, 163, 162.46, 161.94; 209.36, 209.36, 208.63, 207.9, 207.19, 206.48, 205.79, 205.11, 204.45, 203.79, 203.14, 202.5; 251.19, 251.19, 250.33, 249.47, 248.62, 247.79, 246.98, 246.18, 245.39, 244.62, 243.86, 243.12; 293.06, 293.06, 292.07, 291.07, 290.1, 289.14, 288.2, 287.28, 286.38, 285.49, 284.62, 283.77; 334.99, 334.99, 333.86, 332.73, 331.63, 330.54, 329.48, 328.44, 327.41, 326.41, 325.43, 324.46; 377, 377, 375.73, 374.46, 373.22, 372, 370.81, 369.64, 368.5, 367.38, 366.27, 365.19; 419.01, 419.01, 417.69, 416.27, 414.89, 413.54, 412.21, 410.91, 409.64, 408.4, 407.17, 405.98] kJ/kg  cp_TLU_3=[4.2199, 4.2194, 4.1957, 4.1726, 4.1508, 4.13, 4.1103, 4.0916, 4.0738, 4.0569, 4.0408, 4.0254; 4.1955, 4.1951, 4.1769, 4.1592, 4.1422, 4.1259, 4.1103, 4.0954, 4.0812, 4.0676, 4.0545, 4.0421; 4.1843, 4.184, 4.169, 4.1543, 4.1401, 4.1264, 4.1133, 4.1007, 4.0885, 4.0768, 4.0656, 4.0548; 4.1801, 4.1798, 4.1667, 4.1538, 4.1413, 4.1293, 4.1177, 4.1064, 4.0956, 4.0851, 4.075, 4.0653; 4.1796, 4.1794, 4.1675, 4.1558, 4.1444, 4.1334, 4.1227, 4.1123, 4.1023, 4.0926, 4.0832, 4.0741; 4.1813, 4.1813, 4.1702, 4.1592, 4.1484, 4.138, 4.1279, 4.1181, 4.1086, 4.0993, 4.0903, 4.0816; 4.185, 4.185, 4.1742, 4.1636, 4.1532, 4.1432, 4.1334, 4.1239, 4.1146, 4.1056, 4.0969, 4.0884; 4.1901, 4.1901, 4.1795, 4.169, 4.1588, 4.1489, 4.1393, 4.1299, 4.1207, 4.1118, 4.1032, 4.0947; 4.1968, 4.1968, 4.1862, 4.1757, 4.1655, 4.1555, 4.1458, 4.1364, 4.1273, 4.1183, 4.1096, 4.1012; 4.2052, 4.2052, 4.1944, 4.1837, 4.1733, 4.1632, 4.1534, 4.1438, 4.1345, 4.1255, 4.1166, 4.108; 4.2136, 4.2136, 4.2045, 4.1935, 4.1828, 4.1724, 4.1623, 4.1524, 4.1429, 4.1335, 4.1245, 4.1157] kJ/kg/K  u_TLU_4=[.0018; 42.06; 83.948; 125.76; 167.56; 209.36; 251.19; 293.06; 334.99; 377; 418.01] kJ/kg  cp_TLU_5=[4.2199; 4.1955; 4.1843; 4.1801; 4.1796; 4.1813; 4.185; 4.1901; 4.1968; 4.2052; 4.2136] kJ/kg/K  nu_TLU=nu cm^2/s  nu_TLU_2=[1.7917; 1.3061; 1.0032; .8006; .6577; .553; .4739; .4127; .3643; .3254; .2866] mm^2/s  k_TLU=k mW/m/K  k_TLU_2=[561.04; 580.02; 598.44; 615.48; 630.6; 643.61; 654.39; 663.13; 670.02; 675.27; 680.52] mW/m/K
      settings: SourceProductBaseCode=PW,SS,VE
  H1 : PMIOPort  Side=Left
  H2 : PMIOPort  Port=2  Side=Right
  connections:
  Heat Exchanger Characteristic/RConn2 -- Hose Inlet/RConn1 -- Expansion Tank/LConn1
  Heat Exchanger Characteristic/LConn3 -- Sensing Inlet Temperature/RConn1
  Pipe/LConn1 -- Heat Exchanger Characteristic/LConn2
  H1/RConn1 -- Convection Battery-Env/RConn1 -- Heat Exchanger Characteristic/RConn1
  Heat Exchanger Characteristic/LConn1 -- Pipe/LConn2
  Sensing Inlet Temperature/LConn1 -- Pump/RConn1 -- Pipe/RConn1
  Insulator Outlet Hose/LConn1 -- Hose Outlet/LConn2
  Insulator Inlet Hose/LConn1 -- Hose Inlet/LConn2
  " Heat Exchanger Characteristic"/RConn1 -- Convection Battery-Env/LConn1 -- H2/RConn1
  Thermal Liquid Settings (TL)/RConn1 -- Hose Outlet/RConn1 -- Pump/LConn1
  Hose Outlet/LConn1 -- " Heat Exchanger Characteristic"/RConn2
  Sensing Temperature/LConn1 -- Hose Radiator/RConn1 -- Hose Inlet/LConn1
  Hose Radiator/LConn1 -- " Heat Exchanger Characteristic"/LConn2
  " Heat Exchanger Characteristic"/LConn1 -- Hose Radiator/LConn2
  Sensing Temperature/RConn1 -- " Heat Exchanger Characteristic"/LConn3
  PS Terminator/LConn1 -- " Heat Exchanger Characteristic"/RConn3

== system ssc_auto_ev_20b/Step 4: Deployment Model/Thermal @20Hz/Environment ==
  T : Inport
  Ambient Temperature : fl_lib/Thermal/Thermal Sources/Controlled Temperature Source
      settings: SourceProductBaseCode=PW,SS,VE
  Simulink-PS Converter1 : nesl_utility/Simulink-PS Converter  PhysicalDomain=network_engine_domain  SubClassName=ps_input  LeftPortType=input  RightPortType=output  PseudoPeriodic=off  Frequencies=[]  NoiseDistribution=none  NoiseParameters=[]  Unit=degC  AffineConversion=on  FilteringAndDerivatives=zero  SimscapeFilterOrder=1  InputFilterTimeConstant=.001  UdotUserProvided=1
      settings: SourceProductBaseCode=SS,PW,VE
  ThRef1 : fl_lib/Thermal/Thermal Elements/Thermal Reference
      settings: SourceProductBaseCode=PW,SS,VE
  E : PMIOPort  Side=Right
  wires:
  T/1 -> Simulink-PS Converter1/1
  connections:
  Ambient Temperature/LConn1 -- E/RConn1
  Ambient Temperature/RConn1 -- Simulink-PS Converter1/RConn1
  Ambient Temperature/RConn2 -- ThRef1/LConn1

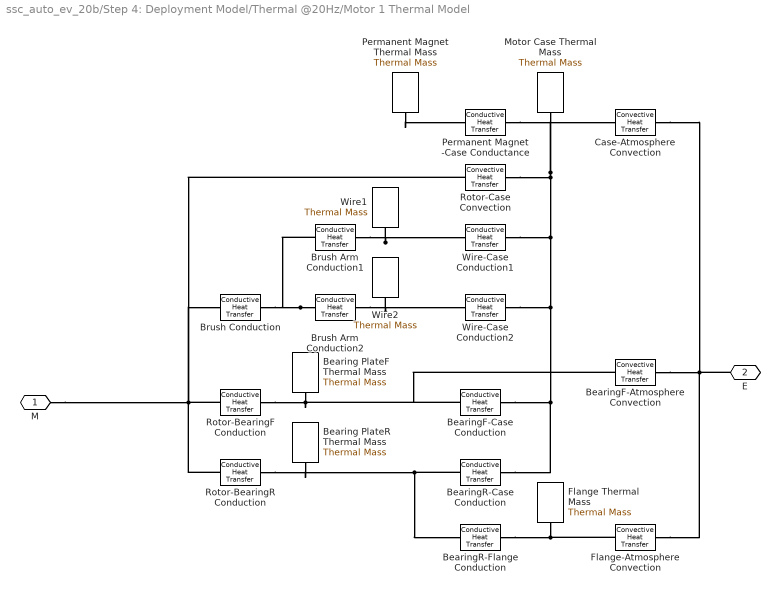
== system ssc_auto_ev_20b/Step 4: Deployment Model/Thermal @20Hz/Motor 1 Thermal Model ==
  Bearing PlateF Thermal Mass : fl_lib/Thermal/Thermal Elements/Thermal Mass  mass=0.6 kg  sp_heat=447 J/kg/K  T_specify=off  T_priority=High  T=300 K  T_nominal_specify=off  T_nominal_unit=K  T_nominal_value=1  Q_specify=off  Q_priority=None  Q=0 W  Q_nominal_specify=off  Q_nominal_unit=W  Q_nominal_value=1
      settings: SourceProductBaseCode=PW,SS,VE
  Bearing PlateR Thermal Mass : fl_lib/Thermal/Thermal Elements/Thermal Mass  mass=0.6 kg  sp_heat=447 J/kg/K  T_specify=off  T_priority=High  T=300 K  T_nominal_specify=off  T_nominal_unit=K  T_nominal_value=1  Q_specify=off  Q_priority=None  Q=0 W  Q_nominal_specify=off  Q_nominal_unit=W  Q_nominal_value=1
      settings: SourceProductBaseCode=PW,SS,VE
  BearingF-Atmosphere Convection : fl_lib/Thermal/Thermal Elements/Convective Heat Transfer  area=274.6 cm^2  heat_tr_coeff=123.5 W/(m^2 * K)  T_specify=off  T_priority=None  T=0 K  T_nominal_specify=off  T_nominal_unit=K  T_nominal_value=1  Q_specify=off  Q_priority=None  Q=0 W  Q_nominal_specify=off  Q_nominal_unit=W  Q_nominal_value=1
      settings: SourceProductBaseCode=PW,SS,VE
  BearingF-Case Conduction : fl_lib/Thermal/Thermal Elements/Conductive Heat Transfer  area=145 cm^2  thickness=18 cm  th_cond=80.2 W/(m*K)  T_specify=off  T_priority=None  T=0 K  T_nominal_specify=off  T_nominal_unit=K  T_nominal_value=1  Q_specify=off  Q_priority=None  Q=0 W  Q_nominal_specify=off  Q_nominal_unit=W  Q_nominal_value=1
      settings: SourceProductBaseCode=PW,SS,VE
  BearingR-Case Conduction : fl_lib/Thermal/Thermal Elements/Conductive Heat Transfer  area=145 cm^2  thickness=25 cm  th_cond=80.2 W/(m*K)  T_specify=off  T_priority=None  T=0 K  T_nominal_specify=off  T_nominal_unit=K  T_nominal_value=1  Q_specify=off  Q_priority=None  Q=0 W  Q_nominal_specify=off  Q_nominal_unit=W  Q_nominal_value=1
      settings: SourceProductBaseCode=PW,SS,VE
  BearingR-Flange Conduction : fl_lib/Thermal/Thermal Elements/Conductive Heat Transfer  area=34.5 cm^2  thickness=14 cm  th_cond=80.2 W/(m*K)  T_specify=off  T_priority=None  T=0 K  T_nominal_specify=off  T_nominal_unit=K  T_nominal_value=1  Q_specify=off  Q_priority=None  Q=0 W  Q_nominal_specify=off  Q_nominal_unit=W  Q_nominal_value=1
      settings: SourceProductBaseCode=PW,SS,VE
  Brush Conduction : fl_lib/Thermal/Thermal Elements/Conductive Heat Transfer  area=3*5 cm^2  thickness=4 cm  th_cond=1.7 W/(m*K)  T_specify=off  T_priority=None  T=0 K  T_nominal_specify=off  T_nominal_unit=K  T_nominal_value=1  Q_specify=off  Q_priority=None  Q=0 W  Q_nominal_specify=off  Q_nominal_unit=W  Q_nominal_value=1
      settings: SourceProductBaseCode=PW,SS,VE
  Brush Arm Conduction1 : fl_lib/Thermal/Thermal Elements/Conductive Heat Transfer  area=3*5 cm^2  thickness=4 cm  th_cond=1.7 W/(m*K)  T_specify=off  T_priority=None  T=0 K  T_nominal_specify=off  T_nominal_unit=K  T_nominal_value=1  Q_specify=off  Q_priority=None  Q=0 W  Q_nominal_specify=off  Q_nominal_unit=W  Q_nominal_value=1
      settings: SourceProductBaseCode=PW,SS,VE
  Brush Arm Conduction2 : fl_lib/Thermal/Thermal Elements/Conductive Heat Transfer  area=3*5 cm^2  thickness=4 cm  th_cond=1.7 W/(m*K)  T_specify=off  T_priority=None  T=0 K  T_nominal_specify=off  T_nominal_unit=K  T_nominal_value=1  Q_specify=off  Q_priority=None  Q=0 W  Q_nominal_specify=off  Q_nominal_unit=W  Q_nominal_value=1
      settings: SourceProductBaseCode=PW,SS,VE
  Case-Atmosphere Convection : fl_lib/Thermal/Thermal Elements/Convective Heat Transfer  area=4240 cm^2  heat_tr_coeff=26.8 W/(m^2 * K)  T_specify=off  T_priority=None  T=0 K  T_nominal_specify=off  T_nominal_unit=K  T_nominal_value=1  Q_specify=off  Q_priority=None  Q=0 W  Q_nominal_specify=off  Q_nominal_unit=W  Q_nominal_value=1
      settings: SourceProductBaseCode=PW,SS,VE
  Flange Thermal Mass : fl_lib/Thermal/Thermal Elements/Thermal Mass  mass=1.6 kg  sp_heat=447 J/kg/K  T_specify=off  T_priority=High  T=300 K  T_nominal_specify=off  T_nominal_unit=K  T_nominal_value=1  Q_specify=off  Q_priority=None  Q=0 W  Q_nominal_specify=off  Q_nominal_unit=W  Q_nominal_value=1
      settings: SourceProductBaseCode=PW,SS,VE
  Flange-Atmosphere Convection : fl_lib/Thermal/Thermal Elements/Convective Heat Transfer  area=324 cm^2  heat_tr_coeff=123.4 W/(m^2 * K)  T_specify=off  T_priority=None  T=0 K  T_nominal_specify=off  T_nominal_unit=K  T_nominal_value=1  Q_specify=off  Q_priority=None  Q=0 W  Q_nominal_specify=off  Q_nominal_unit=W  Q_nominal_value=1
      settings: SourceProductBaseCode=PW,SS,VE
  Motor Case Thermal Mass : fl_lib/Thermal/Thermal Elements/Thermal Mass  mass=3.8 kg  sp_heat=903 J/kg/K  T_specify=off  T_priority=High  T=300 K  T_nominal_specify=off  T_nominal_unit=K  T_nominal_value=1  Q_specify=off  Q_priority=None  Q=0 W  Q_nominal_specify=off  Q_nominal_unit=W  Q_nominal_value=1
      settings: SourceProductBaseCode=PW,SS,VE
  Permanent Magnet Thermal Mass : fl_lib/Thermal/Thermal Elements/Thermal Mass  mass=3.6 kg  sp_heat=447 J/kg/K  T_specify=off  T_priority=High  T=300 K  T_nominal_specify=off  T_nominal_unit=K  T_nominal_value=1  Q_specify=off  Q_priority=None  Q=0 W  Q_nominal_specify=off  Q_nominal_unit=W  Q_nominal_value=1
      settings: SourceProductBaseCode=PW,SS,VE
  Permanent Magnet -Case Conductance : fl_lib/Thermal/Thermal Elements/Conductive Heat Transfer  area=4350 cm^2  thickness=26 cm  th_cond=80.2 W/(m*K)  T_specify=off  T_priority=None  T=0 K  T_nominal_specify=off  T_nominal_unit=K  T_nominal_value=1  Q_specify=off  Q_priority=None  Q=0 W  Q_nominal_specify=off  Q_nominal_unit=W  Q_nominal_value=1
      settings: SourceProductBaseCode=PW,SS,VE
  Rotor-BearingF Conduction : fl_lib/Thermal/Thermal Elements/Conductive Heat Transfer  area=26.4 cm^2  thickness=2.5 cm  th_cond=80.2 W/(m*K)  T_specify=off  T_priority=None  T=0 K  T_nominal_specify=off  T_nominal_unit=K  T_nominal_value=1  Q_specify=off  Q_priority=None  Q=0 W  Q_nominal_specify=off  Q_nominal_unit=W  Q_nominal_value=1
      settings: SourceProductBaseCode=PW,SS,VE
  Rotor-BearingR Conduction : fl_lib/Thermal/Thermal Elements/Conductive Heat Transfer  area=26.4 cm^2  thickness=2.5 cm  th_cond=80.2 W/(m*K)  T_specify=off  T_priority=None  T=0 K  T_nominal_specify=off  T_nominal_unit=K  T_nominal_value=1  Q_specify=off  Q_priority=None  Q=0 W  Q_nominal_specify=off  Q_nominal_unit=W  Q_nominal_value=1
      settings: SourceProductBaseCode=PW,SS,VE
  Rotor-Case Convection : fl_lib/Thermal/Thermal Elements/Convective Heat Transfer  area=1240 cm^2  heat_tr_coeff=210 W/(m^2 * K)  T_specify=off  T_priority=None  T=0 K  T_nominal_specify=off  T_nominal_unit=K  T_nominal_value=1  Q_specify=off  Q_priority=None  Q=0 W  Q_nominal_specify=off  Q_nominal_unit=W  Q_nominal_value=1
      settings: SourceProductBaseCode=PW,SS,VE
  Wire-Case Conduction1 : fl_lib/Thermal/Thermal Elements/Conductive Heat Transfer  area=1 cm^2  thickness=0.2 cm  th_cond=4 W/(m*K)  T_specify=off  T_priority=None  T=0 K  T_nominal_specify=off  T_nominal_unit=K  T_nominal_value=1  Q_specify=off  Q_priority=None  Q=0 W  Q_nominal_specify=off  Q_nominal_unit=W  Q_nominal_value=1
      settings: SourceProductBaseCode=PW,SS,VE
  Wire-Case Conduction2 : fl_lib/Thermal/Thermal Elements/Conductive Heat Transfer  area=1 cm^2  thickness=0.2 cm  th_cond=4 W/(m*K)  T_specify=off  T_priority=None  T=0 K  T_nominal_specify=off  T_nominal_unit=K  T_nominal_value=1  Q_specify=off  Q_priority=None  Q=0 W  Q_nominal_specify=off  Q_nominal_unit=W  Q_nominal_value=1
      settings: SourceProductBaseCode=PW,SS,VE
  Wire1 : fl_lib/Thermal/Thermal Elements/Thermal Mass  mass=0.05 kg  sp_heat=385 J/kg/K  T_specify=off  T_priority=High  T=300 K  T_nominal_specify=off  T_nominal_unit=K  T_nominal_value=1  Q_specify=off  Q_priority=None  Q=0 W  Q_nominal_specify=off  Q_nominal_unit=W  Q_nominal_value=1
      settings: SourceProductBaseCode=PW,SS,VE
  Wire2 : fl_lib/Thermal/Thermal Elements/Thermal Mass  mass=0.05 kg  sp_heat=385 J/kg/K  T_specify=off  T_priority=High  T=300 K  T_nominal_specify=off  T_nominal_unit=K  T_nominal_value=1  Q_specify=off  Q_priority=None  Q=0 W  Q_nominal_specify=off  Q_nominal_unit=W  Q_nominal_value=1
      settings: SourceProductBaseCode=PW,SS,VE
  M : PMIOPort  Side=Right
  E : PMIOPort  Port=2  Side=Left
  connections:
  Wire2/LConn1 -- Wire-Case Conduction2/LConn1 -- Brush Arm Conduction2/RConn1
  Wire1/LConn1 -- Wire-Case Conduction1/LConn1 -- Brush Arm Conduction1/RConn1
  Brush Arm Conduction2/LConn1 -- Brush Arm Conduction1/LConn1 -- Brush Conduction/RConn1
  Permanent Magnet Thermal Mass/LConn1 -- Permanent Magnet -Case Conductance/LConn1
  M/RConn1 -- Rotor-BearingR Conduction/LConn1 -- Rotor-BearingF Conduction/LConn1 -- Brush Conduction/LConn1 -- Rotor-Case Convection/LConn1
  Bearing PlateF Thermal Mass/LConn1 -- Rotor-BearingF Conduction/RConn1 -- BearingF-Atmosphere Convection/LConn1 -- BearingF-Case Conduction/LConn1
  Flange Thermal Mass/LConn1 -- BearingR-Flange Conduction/RConn1 -- Flange-Atmosphere Convection/LConn1
  BearingR-Case Conduction/LConn1 -- BearingR-Flange Conduction/LConn1 -- Bearing PlateR Thermal Mass/LConn1 -- Rotor-BearingR Conduction/RConn1
  Rotor-Case Convection/RConn1 -- BearingR-Case Conduction/RConn1 -- BearingF-Case Conduction/RConn1 -- Wire-Case Conduction2/RConn1 -- Wire-Case Conduction1/RConn1 -- Permanent Magnet -Case Conductance/RConn1 -- Case-Atmosphere Convection/LConn1 -- Motor Case Thermal Mass/LConn1
  Case-Atmosphere Convection/RConn1 -- BearingF-Atmosphere Convection/RConn1 -- E/RConn1 -- Flange-Atmosphere Convection/RConn1
